simulink model "top"  (R2023b)
settings: Solver=VariableStepDiscrete  StartTime=0.0  StopTime=0.12  FixedStep=100e-9  MaxStep=1/120e6  RelTol=1e-3
InitFcn:
  | fw = 50*1e3;
  | Ts = 1/fw;
  | CtrlAPP_m
libraries: spsSeriesRLCBranchLib x11, spsCurrentMeasurementLib x6, spsMosfetLib x5, spsVoltageMeasurementLib x2, spsDCVoltageSourceLib x1, spsPWMGeneratorDCDCLib x1, sps_lib x1
settings Model: Creator=76475  LastModifiedBy=zeus
settings SolverCC: AllowMultiTaskInputOutput=on  ZeroCrossAlgorithm=Adaptive  AutoInsertRateTranBlk=on
settings HardwareCC: ProdBitPerLong=64  ProdHWDeviceType=Intel->x86-64 (Linux 64)
settings ConfigComp: CovScope=ReferencedModels

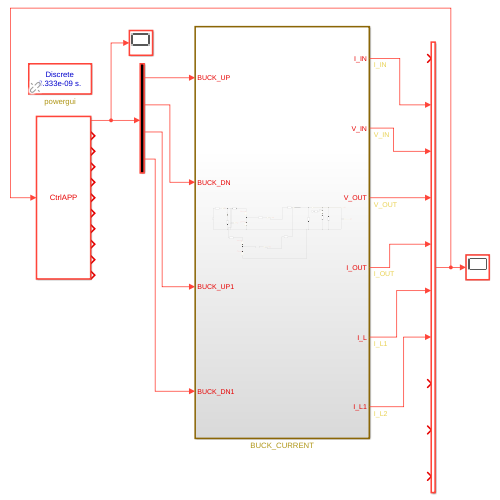
[thumbnail: Simulink's stored preview of the top-level diagram]
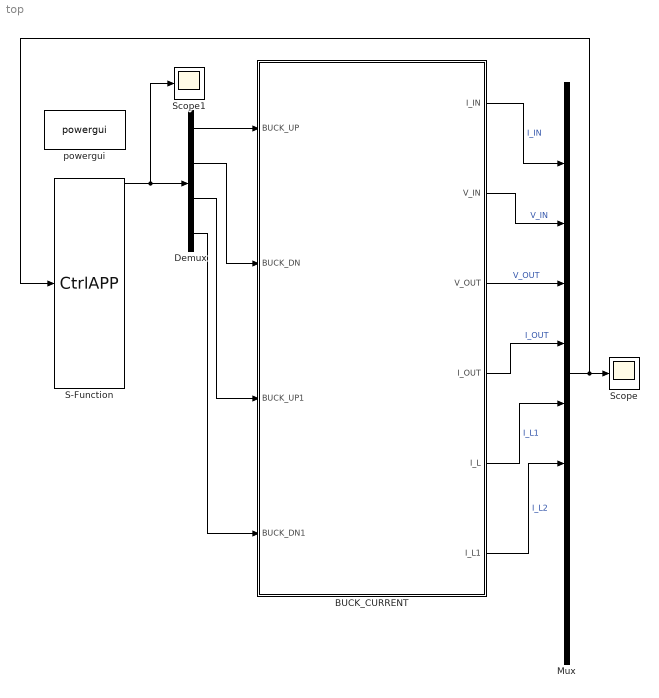
== system top ==
  BUCK_CURRENT : Subsystem
  Demux : Demux
  Mux : Mux  Inputs=10
  S-Function : S-Function  FunctionName=CtrlAPP  SFunctionDeploymentMode=off  EnableBusSupport=off
  Scope : Scope
  Scope1 : Scope
  powergui : sps_lib/powergui  Priority=1  SimulationMode=Discrete  SampleTime=1/120e6  frequency=60  Iterations=50  frequencyindice=0  Pbase=100e6  ErrMax=1e-4  UnitsV=kV  UnitsW=MW  buscounter=0  FunctionMessages=off  echomessages=off  EnableUseOfTLC=off  CurrentSourceSwitches=off  DisableSnubberDevices=off  DisableRonSwitches=off  DisableVfSwitches=off  DisplayEquations=off  AutomaticDiscreteSolvers=off  SolverType=Tustin/Backward Euler (TBE)  Interpol=off  ExternalGateDelay=off  methode=off  Ts=100  x0status=blocks  SPID=on  SwTol=0  HookPort=off  NonlinearTolerance=1e-4  nMaxIteration=100  ContinueOnMaxIteration=off  RestoreLinks=warning  ResistiveCurrentMeasurement=off  Frange=[0:2:500]  Ylog=off  Xlog=on  ShowGrid=off  save=off  variable=ZData  structure=0  ZoomFFT=off  StartTime=0.0  cycles=1  DisplayStyle=1  fundamental=60  FreqAxis=off  MaxFrequency=1000  frequencyindicesteady=1  RmsSteady=1  display=off
  wires:
  BUCK_CURRENT/6(I_L1) -> Mux/7  "I_L2"
  BUCK_CURRENT/4(I_OUT) -> Mux/5  "I_OUT"
  BUCK_CURRENT/2(V_IN) -> Mux/3  "V_IN"
  BUCK_CURRENT/1(I_IN) -> Mux/2  "I_IN"
  Mux/1 -> Scope/1, S-Function/1
  BUCK_CURRENT/3(V_OUT) -> Mux/4  "V_OUT"
  Demux/4 -> BUCK_CURRENT/4(BUCK_DN1)
  Demux/3 -> BUCK_CURRENT/3(BUCK_UP1)
  Demux/2 -> BUCK_CURRENT/2(BUCK_DN)
  Demux/1 -> BUCK_CURRENT/1(BUCK_UP)
  BUCK_CURRENT/5(I_L) -> Mux/6  "I_L1"
  S-Function/1 -> Demux/1, Scope1/1

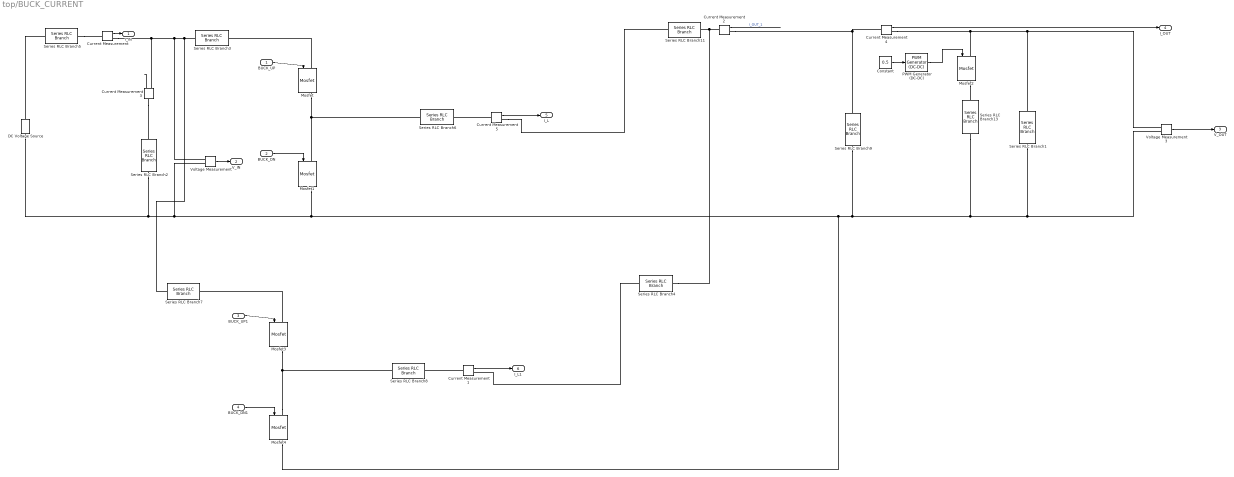
== system top/BUCK_CURRENT ==
  BUCK_UP : Inport
  BUCK_DN : Inport  Port=2
  BUCK_UP1 : Inport  Port=3
  BUCK_DN1 : Inport  Port=4
  Constant : Constant  Value=0.5
  Current Measurement{,1..5} (6 alike) : spsCurrentMeasurementLib/Current Measurement  PhasorSimulation=off  OutputType=Complex  PSBequivalent=0
  DC Voltage Source : spsDCVoltageSourceLib/DC Voltage Source  Amplitude=54  Measurements=None
  Mosfet{,1..4} (5 alike) : spsMosfetLib/Mosfet  Ron=0.01  Lon=0  Rd=0.01  Vfd=0  IC=0  Rs=1e5  Cs=inf  Measurements=on
  PWM Generator (DC-DC) : spsPWMGeneratorDCDCLib/PWM Generator (DC-DC)  Fsw=10  Ts=0
  Series RLC Branch1 : spsSeriesRLCBranchLib/Series RLC Branch  LConnTagsString=__new0  RConnTagsString=__new0  BranchType=R  Resistance=80  Inductance=1e-6  SetiL0=off  InitialCurrent=0  Capacitance=1e-6  Setx0=off  InitialVoltage=0  Measurements=None
  Series RLC Branch11 : spsSeriesRLCBranchLib/Series RLC Branch  LConnTagsString=__new0  RConnTagsString=__new0  BranchType=RL  Resistance=1e-5  Inductance=1e-9  SetiL0=off  InitialCurrent=0  Capacitance=1e-6  Setx0=off  InitialVoltage=0  Measurements=None
  Series RLC Branch13 : spsSeriesRLCBranchLib/Series RLC Branch  LConnTagsString=__new0  RConnTagsString=__new0  BranchType=R  Resistance=0.09  Inductance=1e-6  SetiL0=off  InitialCurrent=0  Capacitance=1e-6  Setx0=off  InitialVoltage=0  Measurements=None
  Series RLC Branch2 : spsSeriesRLCBranchLib/Series RLC Branch  LConnTagsString=__new0  RConnTagsString=__new0  BranchType=RC  Resistance=0.01  Inductance=108e-6  SetiL0=off  InitialCurrent=0  Capacitance=470*4e-6  Setx0=on  InitialVoltage=0  Measurements=None
  Series RLC Branch3 : spsSeriesRLCBranchLib/Series RLC Branch  LConnTagsString=__new0  RConnTagsString=__new0  BranchType=RL  Resistance=1e-5  Inductance=1e-9  SetiL0=off  InitialCurrent=0  Capacitance=1e-6  Setx0=off  InitialVoltage=0  Measurements=None
  Series RLC Branch4 : spsSeriesRLCBranchLib/Series RLC Branch  LConnTagsString=__new0  RConnTagsString=__new0  BranchType=RL  Resistance=1e-5  Inductance=1e-9  SetiL0=off  InitialCurrent=0  Capacitance=1e-6  Setx0=off  InitialVoltage=0  Measurements=None
  Series RLC Branch5 : spsSeriesRLCBranchLib/Series RLC Branch  LConnTagsString=__new0  RConnTagsString=__new0  BranchType=RL  Resistance=1e-3  Inductance=1e-6  SetiL0=off  InitialCurrent=0  Capacitance=1e-6  Setx0=off  InitialVoltage=0  Measurements=None
  Series RLC Branch6 : spsSeriesRLCBranchLib/Series RLC Branch  LConnTagsString=__new0  RConnTagsString=__new0  BranchType=RL  Resistance=0.01  Inductance=10e-6  SetiL0=off  InitialCurrent=0  Capacitance=1e-6  Setx0=off  InitialVoltage=0  Measurements=None
  Series RLC Branch7 : spsSeriesRLCBranchLib/Series RLC Branch  LConnTagsString=__new0  RConnTagsString=__new0  BranchType=RL  Resistance=1e-4  Inductance=1e-8  SetiL0=off  InitialCurrent=0  Capacitance=1e-6  Setx0=off  InitialVoltage=0  Measurements=None
  Series RLC Branch8 : spsSeriesRLCBranchLib/Series RLC Branch  LConnTagsString=__new0  RConnTagsString=__new0  BranchType=RL  Resistance=0.005  Inductance=9.8e-6  SetiL0=off  InitialCurrent=0  Capacitance=1e-6  Setx0=off  InitialVoltage=0  Measurements=None
  Series RLC Branch9 : spsSeriesRLCBranchLib/Series RLC Branch  LConnTagsString=__new0  RConnTagsString=__new0  BranchType=RC  Resistance=0.01  Inductance=108e-6  SetiL0=off  InitialCurrent=0  Capacitance=4000e-6  Setx0=off  InitialVoltage=30  Measurements=None
  Voltage Measurement : spsVoltageMeasurementLib/Voltage Measurement  PhasorSimulation=off  OutputType=Complex  PSBequivalent=0
  Voltage Measurement3 : spsVoltageMeasurementLib/Voltage Measurement  PhasorSimulation=off  OutputType=Complex  PSBequivalent=0
  I_IN : Outport
  V_IN : Outport  Port=2
  V_OUT : Outport  Port=3
  I_OUT : Outport  Port=4
  I_L : Outport  Port=5
  I_L1 : Outport  Port=6
  wires:
  BUCK_UP/1 -> Mosfet/1
  Current Measurement/1 -> I_IN/1
  Voltage Measurement/1 -> V_IN/1
  BUCK_DN/1 -> Mosfet1/1
  Voltage Measurement3/1 -> V_OUT/1
  Current Measurement4/1 -> I_OUT/1
  Current Measurement5/1 -> I_L/1
  Current Measurement2/1 -> ?  "I_OUT_1"
  PWM Generator (DC-DC)/1 -> Mosfet2/1
  Constant/1 -> PWM Generator (DC-DC)/1
  Current Measurement1/1 -> I_L1/1
  BUCK_UP1/1 -> Mosfet3/1
  BUCK_DN1/1 -> Mosfet4/1
  Current Measurement3/1 -> ?
  connections:
  Mosfet/RConn1 -- Series RLC Branch6/LConn1 -- Mosfet1/LConn1
  Mosfet/LConn1 -- Series RLC Branch3/RConn1
  Current Measurement/RConn1 -- Current Measurement3/RConn1 -- Voltage Measurement/LConn1 -- Series RLC Branch7/LConn1 -- Series RLC Branch3/LConn1
  Series RLC Branch5/RConn1 -- Current Measurement/LConn1
  Current Measurement4/LConn1 -- Current Measurement2/RConn1 -- Series RLC Branch9/LConn1
  DC Voltage Source/RConn1 -- Series RLC Branch5/LConn1
  Current Measurement4/RConn1 -- Mosfet2/LConn1 -- Series RLC Branch1/LConn1 -- Voltage Measurement3/LConn1
  Current Measurement5/LConn1 -- Series RLC Branch6/RConn1
  Current Measurement2/LConn1 -- Series RLC Branch4/RConn1 -- Series RLC Branch11/RConn1
  Mosfet2/RConn1 -- Series RLC Branch13/LConn1
  Mosfet4/LConn1 -- Mosfet3/RConn1 -- Series RLC Branch8/LConn1
  Mosfet3/LConn1 -- Series RLC Branch7/RConn1
  Current Measurement1/LConn1 -- Series RLC Branch8/RConn1
  Current Measurement3/LConn1 -- Series RLC Branch2/LConn1
  Current Measurement5/RConn1 -- Series RLC Branch11/LConn1
  Mosfet1/RConn1 -- Mosfet4/RConn1 -- Voltage Measurement3/LConn2 -- Series RLC Branch1/RConn1 -- Series RLC Branch13/RConn1 -- Series RLC Branch9/RConn1 -- DC Voltage Source/LConn1 -- Series RLC Branch2/RConn1 -- Voltage Measurement/LConn2
  Series RLC Branch4/LConn1 -- Current Measurement1/RConn1
